simulink model "esquemaSimulink"  (R2018b)
settings: Solver=VariableStepAuto  StartTime=0.0  StopTime=10.0  RelTol=1e-3
settings Model: Creator=deepin  LastModifiedBy=deepin

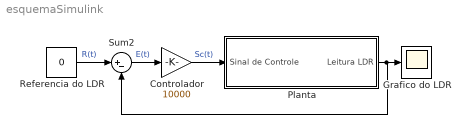
== system esquemaSimulink ==
  Controlador : Gain  Gain=10000
  Grafico do LDR : Scope
  Planta : Subsystem
  Referencia do LDR : Constant  Value=0
  Sum2 : Sum  Inputs=|+-
  wires:
  Sum2/1 -> Controlador/1  "E(t)"
  Planta/1("Leitura LDR ") -> Sum2/2, Grafico do LDR/1
  Referencia do LDR/1 -> Sum2/1  "R(t)"
  Controlador/1 -> Planta/1(Sinal de Controle)  "Sc(t)"

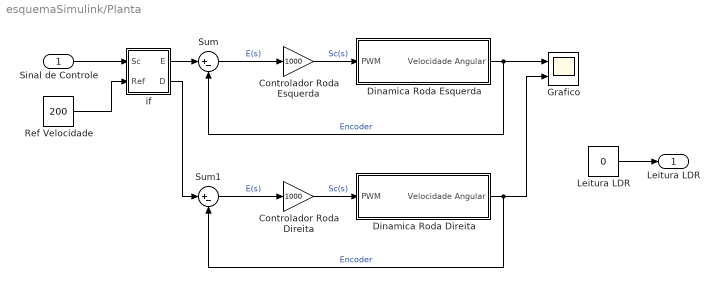
== system esquemaSimulink/Planta ==
  Sinal de Controle : Inport
  Controlador Roda Direita : Gain  Gain=1000
  Controlador Roda Esquerda : Gain  Gain=1000
  Dinamica Roda Direita : Subsystem
  Dinamica Roda Esquerda : Subsystem
  Grafico : Scope  NumInputPorts=2
  Leitura LDR : Constant  Value=0
  Ref Velocidade : Constant  Value=200
  Sum : Sum  Inputs=|+-
  Sum1 : Sum  Inputs=|+-
  if : Subsystem
  "Leitura LDR " : Outport
  wires:
  Dinamica Roda Direita/1(Velocidade Angular) -> Sum1/2, Grafico/2  "Encoder"
  Controlador Roda Direita/1 -> Dinamica Roda Direita/1(PWM)  "Sc(s)"
  Dinamica Roda Esquerda/1(Velocidade Angular) -> Sum/2, Grafico/1  "Encoder"
  Controlador Roda Esquerda/1 -> Dinamica Roda Esquerda/1(PWM)  "Sc(s)"
  Sum1/1 -> Controlador Roda Direita/1  "E(s)"
  Sum/1 -> Controlador Roda Esquerda/1  "E(s)"
  if/1(E) -> Sum/1
  if/2(D) -> Sum1/1
  Sinal de Controle/1 -> if/1(Sc)
  Leitura LDR/1 -> "Leitura LDR "/1
  Ref Velocidade/1 -> if/2(Ref)

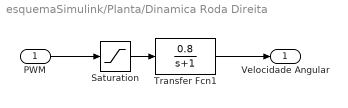
== system esquemaSimulink/Planta/Dinamica Roda Direita ==
  PWM : Inport
  Saturation : Saturate  UpperLimit=255  LowerLimit=-255
  Transfer Fcn1 : TransferFcn  Numerator=[0.8]  Denominator=[1 1]
  Velocidade Angular : Outport
  wires:
  PWM/1 -> Saturation/1
  Transfer Fcn1/1 -> Velocidade Angular/1
  Saturation/1 -> Transfer Fcn1/1

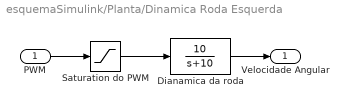
== system esquemaSimulink/Planta/Dinamica Roda Esquerda ==
  PWM : Inport
  Dianamica da roda : TransferFcn  Numerator=[10]  Denominator=[1 10]
  Saturation do PWM : Saturate  UpperLimit=255  LowerLimit=-255
  Velocidade Angular : Outport
  wires:
  Saturation do PWM/1 -> Dianamica da roda/1
  PWM/1 -> Saturation do PWM/1
  Dianamica da roda/1 -> Velocidade Angular/1

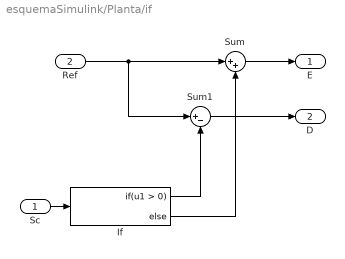
== system esquemaSimulink/Planta/if ==
  Sc : Inport
  Ref : Inport  Port=2
  If : If
  Sum : Sum  Inputs=|++
  Sum1 : Sum  Inputs=|+-
  E : Outport
  D : Outport  Port=2
  wires:
  Ref/1 -> Sum1/1, Sum/1
  Sum/1 -> E/1
  Sum1/1 -> D/1
  Sc/1 -> If/1
  If/1 -> Sum1/2
  If/2 -> Sum/2
